simulink model "k1visetmyt"  (R2015b)
settings: Solver=ode45  StartTime=0.0  StopTime=10.0  RelTol=1e-3
libraries: cdsIPCx x13, cdsCDI64 x4, cdsCDO64 x4, BIO_CD_ENCODE_MASTER x4, BIO_CD_DECODE_MASTER x4, CHK_DIO x4, cdsAdcx0 x1, cdsCDO32 x1, dac x1, TYPEA_MASTER x1, BO_TYPEA_MASTER x1, TESTMON_4CH_MASTER x1
settings Model: Creator=controls  LastModifiedBy=controls
settings DataIOCC: SaveFormat=Array
settings HardwareCC: ProdBitPerPointer=32  ProdLargestAtomicFloat=None  ProdIntDivRoundTo=Undefined  ProdEndianess=Unspecified  ProdWordSize=32  ProdHWDeviceType=32-bit Generic
settings GRTTargetCC: GeneratePreprocessorConditionals=Disable all
settings ConfigComp: CovModelRefEnable=Off

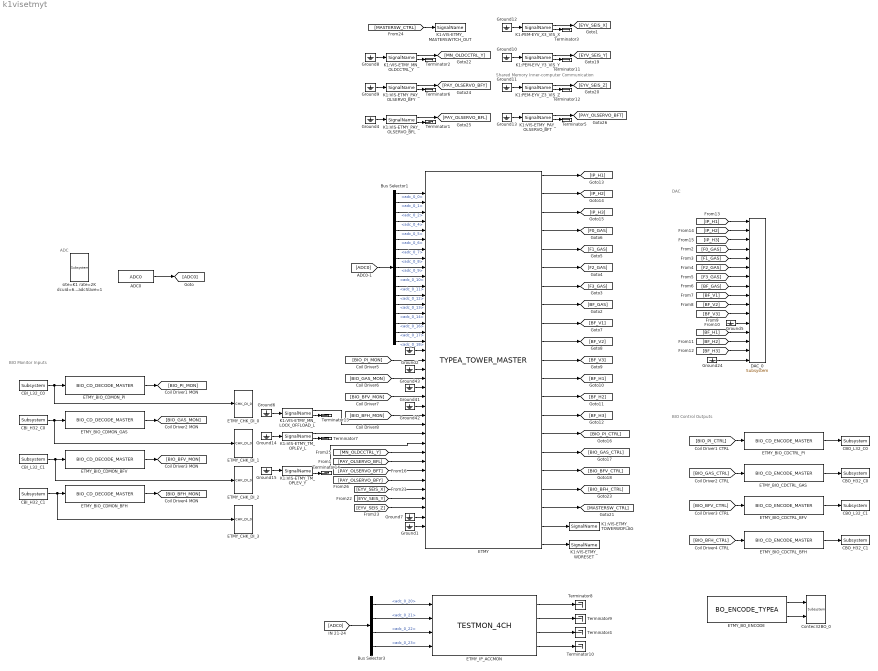
== system k1visetmyt ==
  note: BIO Monitor Inputs
  note: BIO Control Outputs
  note: DAC
  note: ADC
  note: Shared Memory
      | Inner-computer Communication
  ADC0 : cdsAdcx0/ADC0  Tag=cdsAdc  Description=|
      | type-GSC_16AI64SSA
      | card_num=0
      settings: AttributesFormatString=%<Description>\n%<Tag>
  Bus Selector1 : BusSelector  OutputSignals=adc_0_0,adc_0_1,adc_0_2,adc_0_4,adc_0_5,adc_0_6,adc_0_7,adc_0_8,adc_0_9,adc_0_10,adc_0_11,adc_0_12,adc_0_13,adc_0_14,adc_0_16,adc_0_17,adc_0_18
  Bus Selector3 : BusSelector  OutputSignals=adc_0_20,adc_0_21,adc_0_22,adc_0_23
  CBI_H32_C0 : cdsCDI64/Subsystem  Tag=cdsCDI64  Description=card_num=1
      settings: AttributesFormatString=%<Tag>\n%<Description>
  CBI_H32_C1 : cdsCDI64/Subsystem  Tag=cdsCDI64  Description=card_num=3
      settings: AttributesFormatString=%<Tag>\n%<Description>
  CBI_L32_C0 : cdsCDI64/Subsystem  Tag=cdsCDI64  Description=card_num=0
      settings: AttributesFormatString=%<Tag>\n%<Description>
  CBI_L32_C1 : cdsCDI64/Subsystem  Tag=cdsCDI64  Description=card_num=2
      settings: AttributesFormatString=%<Tag>\n%<Description>
  CBO_H32_C0 : cdsCDO64/Subsystem  Tag=cdsCDO64  Description=card_num=1
      settings: AttributesFormatString=%<Tag>\n%<Description>
  CBO_H32_C1 : cdsCDO64/Subsystem  Tag=cdsCDO64  Description=card_num=3
      settings: AttributesFormatString=%<Tag>\n%<Description>
  CBO_L32_C0 : cdsCDO64/Subsystem  Tag=cdsCDO64  Description=card_num=0
      settings: AttributesFormatString=%<Tag>\n%<Description>
  CBO_L32_C1 : cdsCDO64/Subsystem  Tag=cdsCDO64  Description=card_num=2
      settings: AttributesFormatString=%<Tag>\n%<Description>
  Contec32BO_0 : cdsCDO32/Subsystem  Tag=cdsCDO32  Description=Contec32 bit binary output module driver
      settings: AttributesFormatString=%<Tag>
  DAC_0 : dac/Subsystem  Description=|
      | type=GSC_16AO16,
      | card_num=0
      settings: AttributesFormatString=%<Description>
  ETMY : TYPEA_MASTER/TYPEA_TOWER_MASTER
  ETMY_BIO_CDCTRL_BFH : BIO_CD_ENCODE_MASTER/BIO_CD_ENCODE_MASTER
  ETMY_BIO_CDCTRL_BFV : BIO_CD_ENCODE_MASTER/BIO_CD_ENCODE_MASTER
  ETMY_BIO_CDCTRL_GAS : BIO_CD_ENCODE_MASTER/BIO_CD_ENCODE_MASTER
  ETMY_BIO_CDCTRL_PI : BIO_CD_ENCODE_MASTER/BIO_CD_ENCODE_MASTER
  ETMY_BIO_CDMON_BFH : BIO_CD_DECODE_MASTER/BIO_CD_DECODE_MASTER
  ETMY_BIO_CDMON_BFV : BIO_CD_DECODE_MASTER/BIO_CD_DECODE_MASTER
  ETMY_BIO_CDMON_GAS : BIO_CD_DECODE_MASTER/BIO_CD_DECODE_MASTER
  ETMY_BIO_CDMON_PI : BIO_CD_DECODE_MASTER/BIO_CD_DECODE_MASTER
  ETMY_BO_ENCODE : BO_TYPEA_MASTER/BO_ENCODE_TYPEA
  ETMY_CHK_DI_{0..3} (4 alike) : CHK_DIO/CHK_DI_0
  ETMY_IP_ACCMON : TESTMON_4CH_MASTER/TESTMON_4CH
  Ground{1..2,4..15,24,41..43} (18 alike) : Ground
  K1:PEM-EYV_X3_VIS_X : cdsIPCx/SignalName  Tag=cdsIPCx_SHMEM  Description=Inter-Process Communication via Shared memory.
      settings: AttributesFormatString=%<Tag>
  K1:PEM-EYV_Y3_VIS_Y : cdsIPCx/SignalName  Tag=cdsIPCx_SHMEM  Description=Inter-Process Communication via Shared memory.
      settings: AttributesFormatString=%<Tag>
  K1:PEM-EYV_Z3_VIS_Z : cdsIPCx/SignalName  Tag=cdsIPCx_SHMEM  Description=Inter-Process Communication via Shared memory.
      settings: AttributesFormatString=%<Tag>
  K1:VIS-ETMY_MASTERSWITCH_OUT : cdsIPCx/SignalName  Tag=cdsIPCx_SHMEM  Description=Inter-Process Communication via Shared memory.
      settings: AttributesFormatString=%<Tag>
  K1:VIS-ETMY_MN_LOCK_OFFLOAD_L : cdsIPCx/SignalName  Tag=cdsIPCx_SHMEM  Description=Inter-Process Communication via Shared memory.
      settings: AttributesFormatString=%<Tag>
  K1:VIS-ETMY_MN_OLDCCTRL_Y : cdsIPCx/SignalName  Tag=cdsIPCx_SHMEM  Description=Inter-Process Communication via Shared memory.
      settings: AttributesFormatString=%<Tag>
  K1:VIS-ETMY_PAY_OLSERVO_BFL : cdsIPCx/SignalName  Tag=cdsIPCx_SHMEM  Description=Inter-Process Communication via Shared memory.
      settings: AttributesFormatString=%<Tag>
  K1:VIS-ETMY_PAY_OLSERVO_BFT : cdsIPCx/SignalName  Tag=cdsIPCx_SHMEM  Description=Inter-Process Communication via Shared memory.
      settings: AttributesFormatString=%<Tag>
  K1:VIS-ETMY_PAY_OLSERVO_BFY : cdsIPCx/SignalName  Tag=cdsIPCx_SHMEM  Description=Inter-Process Communication via Shared memory.
      settings: AttributesFormatString=%<Tag>
  K1:VIS-ETMY_TM_OPLEV_L : cdsIPCx/SignalName  Tag=cdsIPCx_SHMEM  Description=Inter-Process Communication via Shared memory.
      settings: AttributesFormatString=%<Tag>
  K1:VIS-ETMY_TM_OPLEV_Y : cdsIPCx/SignalName  Tag=cdsIPCx_SHMEM  Description=Inter-Process Communication via Shared memory.
      settings: AttributesFormatString=%<Tag>
  K1:VIS-ETMY_TOWERWDFLAG : cdsIPCx/SignalName  Tag=cdsIPCx_SHMEM  Description=Inter-Process Communication via Shared memory.
      settings: AttributesFormatString=%<Tag>
  K1:VIS-ETMY_WDRESET : cdsIPCx/SignalName  Tag=cdsIPCx_SHMEM  Description=Inter-Process Communication via Shared memory.
      settings: AttributesFormatString=%<Tag>
  Terminator{1..14} (14 alike) : Terminator
  site=K1 rate=2K dcuid=65 host=k1ey1 specific_cpu=5 adcSlave=1 : cdsParameters/Subsystem  Tag=cdsParameters  Description=|
      | Purpose:                                                                                                                                                                                                                                
      | Provide system parameters to the FE code generator to properly configure the generated EPICS names, rep rate of the FE controller, and the Data Acquisition node ID for proper storage of data from this FE controller.                 
      |                                                                                                                                                                                                                                         
      | Useage:                                                                                                                                                                                                                                 
      | The part NAME field is used to identify the FE parameters. It must be of the form:                                                                                                                                                      
      | site=                                                                                                                                                                                                                                   
      | rate=                                                                                                                                                                                                                                   
      | dcuid=                                                                                                                                                                                                                                  
      |                                                                                                                                                                                                                                         
      | Where:                                                                                                                                                                                                                                  
      | site= argument may be H1, H2, L1, M1, G1, either as a single argument or multiple, for example site=H1,H2. These are the only names allowed. These will become the first two characters of all EPICS and signal names (for example G1:).
      |                                                                                                                                                                                                                                         
      | rate= may be 2K, 16K, 32K, or 64K                                                                                                                                                                                                       
      |                                                                                                                                                                                                                                         
      | dcuid= is site specific ie it must be unique at each site.
      settings: AttributesFormatString=%<Tag>
  wires:
  ADC0/1 -> [ADC0]
  ETMY/4 -> [F0_GAS]
  ETMY/5 -> [F1_GAS]
  ETMY/8 -> [BF_GAS]
  ETMY/7 -> [F3_GAS]
  ETMY/6 -> [F2_GAS]
  ETMY/9 -> [BF_V1]
  ETMY/10 -> [BF_V2]
  ETMY/11 -> [BF_V3]
  ETMY/12 -> [BF_H1]
  ETMY/13 -> [BF_H2]
  ETMY/14 -> [BF_H3]
  [BF_H2] -> DAC_0/14
  [BF_V3] -> DAC_0/11
  [BF_H3] -> DAC_0/15
  [BF_V1] -> DAC_0/9
  [BF_H1] -> DAC_0/13
  [BF_V2] -> DAC_0/10
  ETMY/1 -> [IP_H1]
  ETMY/2 -> [IP_H2]
  ETMY/3 -> [IP_H3]
  CBI_H32_C0/1 -> ETMY_CHK_DI_1/1, ETMY_BIO_CDMON_GAS/1
  CBI_L32_C1/1 -> ETMY_CHK_DI_2/1, ETMY_BIO_CDMON_BFV/1
  CBI_L32_C0/1 -> ETMY_CHK_DI_0/1, ETMY_BIO_CDMON_PI/1
  CBI_H32_C1/1 -> ETMY_CHK_DI_3/1, ETMY_BIO_CDMON_BFH/1
  ETMY_BIO_CDCTRL_BFH/1 -> CBO_H32_C1/1
  ETMY_BIO_CDCTRL_PI/1 -> CBO_L32_C0/1
  ETMY_BIO_CDCTRL_GAS/1 -> CBO_H32_C0/1
  ETMY_BIO_CDCTRL_BFV/1 -> CBO_L32_C1/1
  [BIO_PI_CTRL] -> ETMY_BIO_CDCTRL_PI/1
  [BIO_GAS_CTRL] -> ETMY_BIO_CDCTRL_GAS/1
  [BIO_BFV_CTRL] -> ETMY_BIO_CDCTRL_BFV/1
  ETMY_BIO_CDMON_PI/1 -> [BIO_PI_MON]
  ETMY_BIO_CDMON_GAS/1 -> [BIO_GAS_MON]
  ETMY_BIO_CDMON_BFH/1 -> [BIO_BFH_MON]
  ETMY_BIO_CDMON_BFV/1 -> [BIO_BFV_MON]
  [BIO_BFH_CTRL] -> ETMY_BIO_CDCTRL_BFH/1
  [IP_H1] -> DAC_0/1
  [IP_H2] -> DAC_0/2
  [IP_H3] -> DAC_0/3
  [F0_GAS] -> DAC_0/4
  [F1_GAS] -> DAC_0/5
  [F2_GAS] -> DAC_0/6
  [F3_GAS] -> DAC_0/7
  [BF_GAS] -> DAC_0/8
  [ADC0] -> Bus Selector3/1
  Bus Selector3/2 -> ETMY_IP_ACCMON/2  "<adc_0_21>"
  Bus Selector3/1 -> ETMY_IP_ACCMON/1  "<adc_0_20>"
  Bus Selector3/3 -> ETMY_IP_ACCMON/3  "<adc_0_22>"
  Bus Selector3/4 -> ETMY_IP_ACCMON/4  "<adc_0_23>"
  ETMY_IP_ACCMON/3 -> Terminator4/1
  ETMY_IP_ACCMON/4 -> Terminator10/1
  ETMY_IP_ACCMON/1 -> Terminator8/1
  ETMY_IP_ACCMON/2 -> Terminator9/1
  Ground5/1 -> DAC_0/12
  Ground24/1 -> DAC_0/16
  ETMY/15 -> [BIO_PI_CTRL]
  ETMY/16 -> [BIO_GAS_CTRL]
  ETMY/17 -> [BIO_BFV_CTRL]
  ETMY/18 -> [BIO_BFH_CTRL]
  ETMY_BO_ENCODE/1 -> Contec32BO_0/1
  ETMY_BO_ENCODE/2 -> Contec32BO_0/2
  [ADC0] -> Bus Selector1/1
  Bus Selector1/1 -> ETMY/1  "<adc_0_0>"
  Bus Selector1/2 -> ETMY/2  "<adc_0_1>"
  Bus Selector1/3 -> ETMY/3  "<adc_0_2>"
  Bus Selector1/4 -> ETMY/4  "<adc_0_4>"
  Bus Selector1/5 -> ETMY/5  "<adc_0_5>"
  Bus Selector1/6 -> ETMY/6  "<adc_0_6>"
  Bus Selector1/7 -> ETMY/7  "<adc_0_7>"
  Bus Selector1/8 -> ETMY/8  "<adc_0_8>"
  Bus Selector1/9 -> ETMY/9  "<adc_0_9>"
  Bus Selector1/10 -> ETMY/10  "<adc_0_10>"
  Bus Selector1/11 -> ETMY/11  "<adc_0_11>"
  Bus Selector1/12 -> ETMY/12  "<adc_0_12>"
  Bus Selector1/13 -> ETMY/13  "<adc_0_13>"
  Bus Selector1/14 -> ETMY/14  "<adc_0_14>"
  Bus Selector1/15 -> ETMY/15  "<adc_0_16>"
  Bus Selector1/16 -> ETMY/16  "<adc_0_17>"
  Bus Selector1/17 -> ETMY/17  "<adc_0_18>"
  [BIO_PI_MON] -> ETMY/19
  [BIO_GAS_MON] -> ETMY/21
  [BIO_BFV_MON] -> ETMY/23
  [BIO_BFH_MON] -> ETMY/25
  Ground43/1 -> ETMY/20
  Ground41/1 -> ETMY/22
  Ground42/1 -> ETMY/24
  Ground2/1 -> ETMY/18
  Ground12/1 -> K1:PEM-EYV_X3_VIS_X/1
  K1:PEM-EYV_X3_VIS_X/2 -> Terminator3/1
  Ground10/1 -> K1:PEM-EYV_Y3_VIS_Y/1
  K1:PEM-EYV_Y3_VIS_Y/2 -> Terminator11/1
  Ground11/1 -> K1:PEM-EYV_Z3_VIS_Z/1
  K1:PEM-EYV_Z3_VIS_Z/2 -> Terminator12/1
  K1:PEM-EYV_X3_VIS_X/1 -> [EYV_SEIS_X]
  K1:PEM-EYV_Y3_VIS_Y/1 -> [EYV_SEIS_Y]
  K1:PEM-EYV_Z3_VIS_Z/1 -> [EYV_SEIS_Z]
  K1:VIS-ETMY_PAY_OLSERVO_BFY/2 -> Terminator6/1
  K1:VIS-ETMY_MN_OLDCCTRL_Y/2 -> Terminator2/1
  Ground8/1 -> K1:VIS-ETMY_MN_OLDCCTRL_Y/1
  Ground9/1 -> K1:VIS-ETMY_PAY_OLSERVO_BFY/1
  K1:VIS-ETMY_MN_OLDCCTRL_Y/1 -> [MN_OLDCCTRL_Y]
  K1:VIS-ETMY_PAY_OLSERVO_BFY/1 -> [PAY_OLSERVO_BFY]
  K1:VIS-ETMY_PAY_OLSERVO_BFL/2 -> Terminator1/1
  Ground4/1 -> K1:VIS-ETMY_PAY_OLSERVO_BFL/1
  K1:VIS-ETMY_PAY_OLSERVO_BFL/1 -> [PAY_OLSERVO_BFL]
  K1:VIS-ETMY_PAY_OLSERVO_BFT/2 -> Terminator5/1
  Ground13/1 -> K1:VIS-ETMY_PAY_OLSERVO_BFT/1
  K1:VIS-ETMY_PAY_OLSERVO_BFT/1 -> [PAY_OLSERVO_BFT]
  Ground14/1 -> K1:VIS-ETMY_TM_OPLEV_L/1
  K1:VIS-ETMY_TM_OPLEV_L/2 -> Terminator7/1
  Ground15/1 -> K1:VIS-ETMY_TM_OPLEV_Y/1
  K1:VIS-ETMY_TM_OPLEV_Y/2 -> Terminator14/1
  ETMY/20 -> K1:VIS-ETMY_TOWERWDFLAG/1
  ETMY/21 -> K1:VIS-ETMY_WDRESET/1
  ETMY/19 -> [MASTERSW_CTRL]
  [MASTERSW_CTRL] -> K1:VIS-ETMY_MASTERSWITCH_OUT/1
  K1:VIS-ETMY_MN_LOCK_OFFLOAD_L/1 -> ETMY/26
  Ground1/1 -> ETMY/37
  Ground7/1 -> ETMY/36
  [PAY_OLSERVO_BFL] -> ETMY/30
  [EYV_SEIS_X] -> ETMY/33
  [EYV_SEIS_Y] -> ETMY/34
  [EYV_SEIS_Z] -> ETMY/35
  [MN_OLDCCTRL_Y] -> ETMY/29
  [PAY_OLSERVO_BFY] -> ETMY/32
  [PAY_OLSERVO_BFT] -> ETMY/31
  K1:VIS-ETMY_TM_OPLEV_Y/1 -> ETMY/28
  K1:VIS-ETMY_TM_OPLEV_L/1 -> ETMY/27
  Ground6/1 -> K1:VIS-ETMY_MN_LOCK_OFFLOAD_L/1
  K1:VIS-ETMY_MN_LOCK_OFFLOAD_L/2 -> Terminator13/1
